simulink model "Bicopter"  (R2025a)
settings: Solver=VariableStepAuto  StartTime=0.0  StopTime=10.0  RelTol=1e-3
values from neighbouring files (symbols this model uses):
  g = 9.81    [biCopter_Variable_script.m]
  initial_states = [initial_position; initial_angles; initial_velocity; initial_ang_velocity]    [biCopter_Variable_script.m]
  Ixx = 0.005    [biCopter_Variable_script.m]
  Iyy = 0.005    [biCopter_Variable_script.m]
  Izz = 0.01    [biCopter_Variable_script.m]
  k_T = 1.5e-6    (= 1.5e-06)    [biCopter_Variable_script.m]
  L = 0.25    [biCopter_Variable_script.m]
  m = 0.5    [biCopter_Variable_script.m]
  max_servo_angle = pi/6    (= 0.523598775598)    [biCopter_Variable_script.m]
  max_thrust_per_motor = 5    [biCopter_Variable_script.m]
  min_servo_angle = -pi/6    (= -0.523598775598)    [biCopter_Variable_script.m]
  min_thrust_per_motor = 0    [biCopter_Variable_script.m]
  tau_motor = 0.05    [biCopter_Variable_script.m]
libraries: slpidlib x4
settings Model: Creator=adity  LastModifiedBy=adity

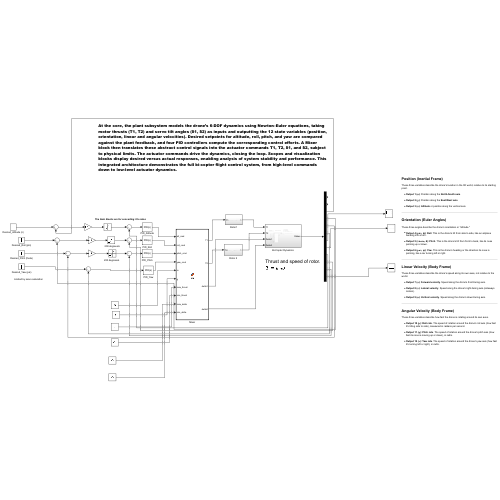
[thumbnail: Simulink's stored preview of the top-level diagram]
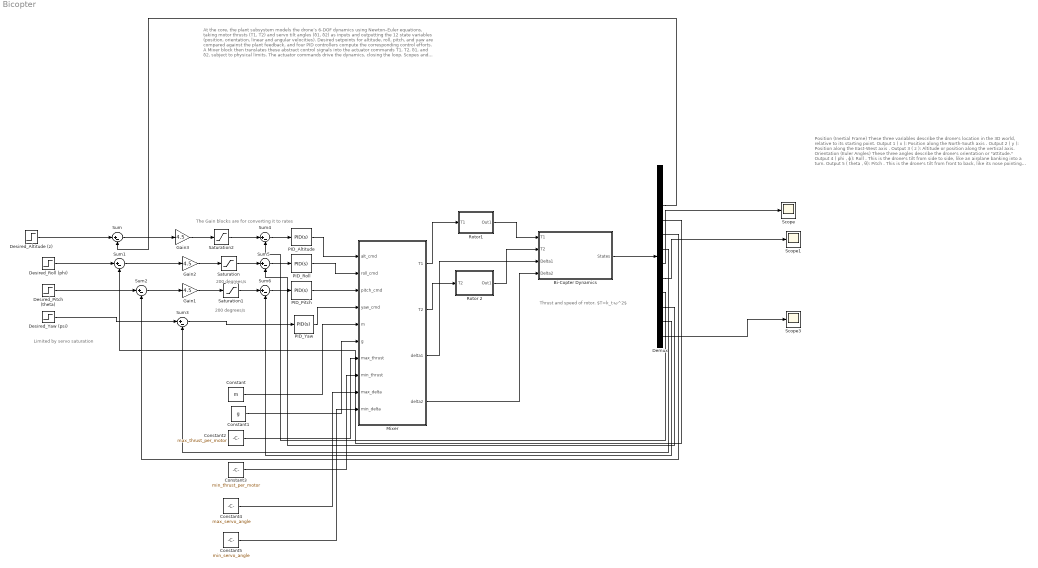
== system Bicopter ==
  note: Limited by servo saturation
  note: 200 degrees/s
  note: The Gain blocks are for converting it to rates
  note: Position (Inertial Frame)
      | These three variables describe the drone's location in the 3D world, relative to its starting point.
      | Output 1 ( x ): Position along the North-South axis .
      | Output 2 ( y ): Position along the East-West axis .
      | Output 3 ( z ): Altitude or position along the vertical axis.
      | Orientation (Euler Angles)
      | These three angles describe the drone's orientation or "attitude."
      | Output 4 ( phi , ϕ): Roll . This is the drone's tilt from side to side, like an airplane banking into a turn.
      | Output 5 ( theta , θ): Pitch . This is the drone's tilt from front to back, like its nose pointing up or down.
      | Output 6 ( psi , ψ): Yaw . This is the drone's heading or the direction its nose is pointing, like a car turning left or right.
      | Linear Velocity (Body Frame)
      | These three variables describe the drone's speed along its own axes, not relative to the world.
      | Output 7 ( u ): Forward velocity . Speed along the drone's front-facing axis.
      | Output 8 ( v ): Lateral velocity . Speed along the drone's right-facing axis (sideways motion).
      | Output 9 ( w ): Vertical velocity . Speed along the drone's down-facing axis.
      | Angular Velocity (Body Frame)
      | These three variables describe how fast the drone is rotating around its own axes.
      | Output 10 ( p ): Roll rate . The speed of rotation around the drone's roll axis (how fast it's tilting side to side), measured in radians per second.
      | Output 11 ( q ): Pitch rate . The speed of rotation around the drone's pitch axis (how fast its nose is moving up or down), in rad/s.
      | Output 12 ( r ): Yaw rate . The speed of rotation around the drone's yaw axis (how fast it's turning left or right), in rad/s.
  note: Thrust and speed of rotor.
      | $T=k_t​⋅ω^2$
  note: At the core, the plant subsystem models the drone’s 6-DOF dynamics using Newton–Euler equations, taking motor thrusts (T1, T2) and servo tilt angles (δ1, δ2) as inputs and outputting the 12 state variables (position, orientation, linear and angular velocities). Desired setpoints for altitude, roll, pitch, and yaw are compared against the plant feedback, and four PID controllers compute the corresponding control efforts. A Mixer block then translates these abstract control signals into the actuator commands T1, T2, δ1, and δ2, subject to physical limits. The actuator commands drive the dynamics, closing the loop. Scopes and visualization blocks display desired versus actual responses, enabling analysis of system stability and performance. This integrated architecture demonstrates the full bi-copter flight control system, from high-level commands down to low-level actuator dynamics.
  note: 200 degrees/s
  Bi-Copter Dynamics : Subsystem
  Constant : Constant  Value=m
  Constant1 : Constant  Value=g
  Constant2 : Constant  Value=max_thrust_per_motor
  Constant3 : Constant  Value=min_thrust_per_motor
  Constant4 : Constant  Value=max_servo_angle
  Constant5 : Constant  Value=min_servo_angle
  Demux : Demux  Outputs=12
  Desired_Altitude (z) : Step  Time=0  After=500  SampleTime=0
  Desired_Pitch (theta) : Step  Time=0  After=0.5  SampleTime=0
  Desired_Roll (phi) : Step  Time=0  After=10  SampleTime=0
  Desired_Yaw (psi) : Step  Time=0  After=2.3  SampleTime=0
  Gain1 : Gain  Gain=4.5
  Gain2 : Gain  Gain=4.5
  Gain3 : Gain  Gain=4.5
  Mixer : MATLAB Function  TreatAsAtomicUnit=on
  PID_Altitude : slpidlib/PID Controller  Controller=PID  Form=Parallel  TimeDomain=Continuous-time  UseExternalTs=off  SampleTime=-1  IntegratorMethod=Forward Euler  FilterMethod=Forward Euler  ControllerParametersSource=internal  P=1  I=1  UseKiTs=off  D=0  UseExternalDerivativeSource=off  N=100  UseFilter=on  TunerSelectOption=Transfer Function Based (PID Tuner App)  InitialConditionSource=internal  InitialConditionForIntegrator=0  InitialConditionForFilter=0  DifferentiatorICPrevScaledInput=0  ExternalReset=none  TrackingMode=off  Kt=1  LimitOutput=off  SatLimitsSource=internal  UpperSaturationLimit=inf  LowerSaturationLimit=-inf  LinearizeAsGain=on  AntiWindupMode=none  Kb=1  LimitIntegrator=off  UpperIntegratorSaturationLimit=inf  LowerIntegratorSaturationLimit=-inf  POutMin=[]  POutMax=[]  IOutMin=[]  IOutMax=[]  DOutMin=[]  DOutMax=[]  NOutMin=[]  NOutMax=[]  SumOutMin=[]  SumOutMax=[]  SaturationOutMin=[]  SaturationOutMax=[]  PParamMin=[]  PParamMax=[]  IParamMin=[]  IParamMax=[]  DParamMin=[]  DParamMax=[]  NParamMin=[]  NParamMax=[]  KbParamMin=[]  KbParamMax=[]  KtParamMin=[]  KtParamMax=[]  KbOutMin=[]  KbOutMax=[]  KtOutMin=[]  KtOutMax=[]  IntegratorOutMin=[]  IntegratorOutMax=[]  FilterOutMin=[]  FilterOutMax=[]  SumI1OutMin=[]  SumI1OutMax=[]  SumI2OutMin=[]  SumI2OutMax=[]  SumI3OutMin=[]  SumI3OutMax=[]  SumI4OutMin=[]  SumI4OutMax=[]  SumDOutMin=[]  SumDOutMax=[]  DifferentiatorOutMin=[]  DifferentiatorOutMax=[]  FilterDiffOutCoefMin=[]  FilterDiffOutCoefMax=[]  ReciprocalOutMin=[]  ReciprocalOutMax=[]  SumDenOutMin=[]  SumDenOutMax=[]  SumNumOutMin=[]  SumNumOutMax=[]  DivideOutMin=[]  DivideOutMax=[]  UdiffTsProdOutMin=[]  UdiffTsProdOutMax=[]  NTsProdOutMin=[]  NTsProdOutMax=[]  UintegralTsProdOutMin=[]  UintegralTsProdOutMax=[]  UngainTsProdOutMin=[]  UngainTsProdOutMax=[]  ClampingZeroOutDataTypeStr=Inherit: Inherit via back propagation  ClampingZeroOutMin=[]  ClampingZeroOutMax=[]  FilterDenConstantOutDataTypeStr=Inherit: Inherit via back propagation  FilterDenConstantOutMin=[]  FilterDenConstantOutMax=[]  PCopyOutDataTypeStr=Inherit: Inherit via back propagation  PCopyOutMin=[]  PCopyOutMax=[]  NCopyOutDataTypeStr=Inherit: Inherit via back propagation  NCopyOutMin=[]  NCopyOutMax=[]  IntegratorContinuousStateAttributes=''  IntegratorStateMustResolveToSignalObject=off  IntegratorRTWStateStorageClass=Auto  FilterContinuousStateAttributes=''  FilterStateMustResolveToSignalObject=off  FilterRTWStateStorageClass=Auto  ParallelPVariant=InternalParameters  IdealPVariant=Disabled  IVariant=InternalParameters  DVariant=InternalParameters  IntegratorVariant=Continuous  SatVariant=Disabled  AWVariant=Passthrough  PCopyVariant=Disabled  TRVariant=Disabled  FdbkBlocksVariant=Forward  IdealPFdbkVariant=Disabled  SatFdbkVariant=Disabled  DerivativeFilterVariant=ContFilter  NVariant=InternalParameters  NCopyVariant=Disabled  FilterICVariant=InternalICsFilter  IntegratorICVariant=InternalICs  ExternalResetVariant=Disabled  TRSumVariant=Passthrough  SumFdbkVariant=Disabled  SumVariant=Sum_PID  TsampFilterVariant=InternalTs  TsampNgainVariant=Passthrough  TsampIntegralVariant=Disabled_SignalSpec  ExternalSaturationOutDataTypeStr=Inherit: Same as second input  DerivativeSourceVariant=ErrorSignal  PreIntVariant=InternalPreInt
  PID_Pitch : slpidlib/PID Controller  Controller=PID  Form=Parallel  TimeDomain=Continuous-time  UseExternalTs=off  SampleTime=-1  IntegratorMethod=Forward Euler  FilterMethod=Forward Euler  ControllerParametersSource=internal  P=1  I=1  UseKiTs=off  D=0  UseExternalDerivativeSource=off  N=100  UseFilter=on  TunerSelectOption=Transfer Function Based (PID Tuner App)  InitialConditionSource=internal  InitialConditionForIntegrator=0  InitialConditionForFilter=0  DifferentiatorICPrevScaledInput=0  ExternalReset=none  TrackingMode=off  Kt=1  LimitOutput=off  SatLimitsSource=internal  UpperSaturationLimit=inf  LowerSaturationLimit=-inf  LinearizeAsGain=on  AntiWindupMode=none  Kb=1  LimitIntegrator=off  UpperIntegratorSaturationLimit=inf  LowerIntegratorSaturationLimit=-inf  POutMin=[]  POutMax=[]  IOutMin=[]  IOutMax=[]  DOutMin=[]  DOutMax=[]  NOutMin=[]  NOutMax=[]  SumOutMin=[]  SumOutMax=[]  SaturationOutMin=[]  SaturationOutMax=[]  PParamMin=[]  PParamMax=[]  IParamMin=[]  IParamMax=[]  DParamMin=[]  DParamMax=[]  NParamMin=[]  NParamMax=[]  KbParamMin=[]  KbParamMax=[]  KtParamMin=[]  KtParamMax=[]  KbOutMin=[]  KbOutMax=[]  KtOutMin=[]  KtOutMax=[]  IntegratorOutMin=[]  IntegratorOutMax=[]  FilterOutMin=[]  FilterOutMax=[]  SumI1OutMin=[]  SumI1OutMax=[]  SumI2OutMin=[]  SumI2OutMax=[]  SumI3OutMin=[]  SumI3OutMax=[]  SumI4OutMin=[]  SumI4OutMax=[]  SumDOutMin=[]  SumDOutMax=[]  DifferentiatorOutMin=[]  DifferentiatorOutMax=[]  FilterDiffOutCoefMin=[]  FilterDiffOutCoefMax=[]  ReciprocalOutMin=[]  ReciprocalOutMax=[]  SumDenOutMin=[]  SumDenOutMax=[]  SumNumOutMin=[]  SumNumOutMax=[]  DivideOutMin=[]  DivideOutMax=[]  UdiffTsProdOutMin=[]  UdiffTsProdOutMax=[]  NTsProdOutMin=[]  NTsProdOutMax=[]  UintegralTsProdOutMin=[]  UintegralTsProdOutMax=[]  UngainTsProdOutMin=[]  UngainTsProdOutMax=[]  ClampingZeroOutDataTypeStr=Inherit: Inherit via back propagation  ClampingZeroOutMin=[]  ClampingZeroOutMax=[]  FilterDenConstantOutDataTypeStr=Inherit: Inherit via back propagation  FilterDenConstantOutMin=[]  FilterDenConstantOutMax=[]  PCopyOutDataTypeStr=Inherit: Inherit via back propagation  PCopyOutMin=[]  PCopyOutMax=[]  NCopyOutDataTypeStr=Inherit: Inherit via back propagation  NCopyOutMin=[]  NCopyOutMax=[]  IntegratorContinuousStateAttributes=''  IntegratorStateMustResolveToSignalObject=off  IntegratorRTWStateStorageClass=Auto  FilterContinuousStateAttributes=''  FilterStateMustResolveToSignalObject=off  FilterRTWStateStorageClass=Auto  ParallelPVariant=InternalParameters  IdealPVariant=Disabled  IVariant=InternalParameters  DVariant=InternalParameters  IntegratorVariant=Continuous  SatVariant=Disabled  AWVariant=Passthrough  PCopyVariant=Disabled  TRVariant=Disabled  FdbkBlocksVariant=Forward  IdealPFdbkVariant=Disabled  SatFdbkVariant=Disabled  DerivativeFilterVariant=ContFilter  NVariant=InternalParameters  NCopyVariant=Disabled  FilterICVariant=InternalICsFilter  IntegratorICVariant=InternalICs  ExternalResetVariant=Disabled  TRSumVariant=Passthrough  SumFdbkVariant=Disabled  SumVariant=Sum_PID  TsampFilterVariant=InternalTs  TsampNgainVariant=Passthrough  TsampIntegralVariant=Disabled_SignalSpec  ExternalSaturationOutDataTypeStr=Inherit: Same as second input  DerivativeSourceVariant=ErrorSignal  PreIntVariant=InternalPreInt
  PID_Roll : slpidlib/PID Controller  Controller=PID  Form=Parallel  TimeDomain=Continuous-time  UseExternalTs=off  SampleTime=-1  IntegratorMethod=Forward Euler  FilterMethod=Forward Euler  ControllerParametersSource=internal  P=1  I=1  UseKiTs=off  D=0  UseExternalDerivativeSource=off  N=100  UseFilter=on  TunerSelectOption=Transfer Function Based (PID Tuner App)  InitialConditionSource=internal  InitialConditionForIntegrator=0  InitialConditionForFilter=0  DifferentiatorICPrevScaledInput=0  ExternalReset=none  TrackingMode=off  Kt=1  LimitOutput=off  SatLimitsSource=internal  UpperSaturationLimit=inf  LowerSaturationLimit=-inf  LinearizeAsGain=on  AntiWindupMode=none  Kb=1  LimitIntegrator=off  UpperIntegratorSaturationLimit=inf  LowerIntegratorSaturationLimit=-inf  POutMin=[]  POutMax=[]  IOutMin=[]  IOutMax=[]  DOutMin=[]  DOutMax=[]  NOutMin=[]  NOutMax=[]  SumOutMin=[]  SumOutMax=[]  SaturationOutMin=[]  SaturationOutMax=[]  PParamMin=[]  PParamMax=[]  IParamMin=[]  IParamMax=[]  DParamMin=[]  DParamMax=[]  NParamMin=[]  NParamMax=[]  KbParamMin=[]  KbParamMax=[]  KtParamMin=[]  KtParamMax=[]  KbOutMin=[]  KbOutMax=[]  KtOutMin=[]  KtOutMax=[]  IntegratorOutMin=[]  IntegratorOutMax=[]  FilterOutMin=[]  FilterOutMax=[]  SumI1OutMin=[]  SumI1OutMax=[]  SumI2OutMin=[]  SumI2OutMax=[]  SumI3OutMin=[]  SumI3OutMax=[]  SumI4OutMin=[]  SumI4OutMax=[]  SumDOutMin=[]  SumDOutMax=[]  DifferentiatorOutMin=[]  DifferentiatorOutMax=[]  FilterDiffOutCoefMin=[]  FilterDiffOutCoefMax=[]  ReciprocalOutMin=[]  ReciprocalOutMax=[]  SumDenOutMin=[]  SumDenOutMax=[]  SumNumOutMin=[]  SumNumOutMax=[]  DivideOutMin=[]  DivideOutMax=[]  UdiffTsProdOutMin=[]  UdiffTsProdOutMax=[]  NTsProdOutMin=[]  NTsProdOutMax=[]  UintegralTsProdOutMin=[]  UintegralTsProdOutMax=[]  UngainTsProdOutMin=[]  UngainTsProdOutMax=[]  ClampingZeroOutDataTypeStr=Inherit: Inherit via back propagation  ClampingZeroOutMin=[]  ClampingZeroOutMax=[]  FilterDenConstantOutDataTypeStr=Inherit: Inherit via back propagation  FilterDenConstantOutMin=[]  FilterDenConstantOutMax=[]  PCopyOutDataTypeStr=Inherit: Inherit via back propagation  PCopyOutMin=[]  PCopyOutMax=[]  NCopyOutDataTypeStr=Inherit: Inherit via back propagation  NCopyOutMin=[]  NCopyOutMax=[]  IntegratorContinuousStateAttributes=''  IntegratorStateMustResolveToSignalObject=off  IntegratorRTWStateStorageClass=Auto  FilterContinuousStateAttributes=''  FilterStateMustResolveToSignalObject=off  FilterRTWStateStorageClass=Auto  ParallelPVariant=InternalParameters  IdealPVariant=Disabled  IVariant=InternalParameters  DVariant=InternalParameters  IntegratorVariant=Continuous  SatVariant=Disabled  AWVariant=Passthrough  PCopyVariant=Disabled  TRVariant=Disabled  FdbkBlocksVariant=Forward  IdealPFdbkVariant=Disabled  SatFdbkVariant=Disabled  DerivativeFilterVariant=ContFilter  NVariant=InternalParameters  NCopyVariant=Disabled  FilterICVariant=InternalICsFilter  IntegratorICVariant=InternalICs  ExternalResetVariant=Disabled  TRSumVariant=Passthrough  SumFdbkVariant=Disabled  SumVariant=Sum_PID  TsampFilterVariant=InternalTs  TsampNgainVariant=Passthrough  TsampIntegralVariant=Disabled_SignalSpec  ExternalSaturationOutDataTypeStr=Inherit: Same as second input  DerivativeSourceVariant=ErrorSignal  PreIntVariant=InternalPreInt
  PID_Yaw : slpidlib/PID Controller  Controller=PID  Form=Parallel  TimeDomain=Continuous-time  UseExternalTs=off  SampleTime=-1  IntegratorMethod=Forward Euler  FilterMethod=Forward Euler  ControllerParametersSource=internal  P=1  I=1  UseKiTs=off  D=0  UseExternalDerivativeSource=off  N=100  UseFilter=on  TunerSelectOption=Transfer Function Based (PID Tuner App)  InitialConditionSource=internal  InitialConditionForIntegrator=0  InitialConditionForFilter=0  DifferentiatorICPrevScaledInput=0  ExternalReset=none  TrackingMode=off  Kt=1  LimitOutput=off  SatLimitsSource=internal  UpperSaturationLimit=inf  LowerSaturationLimit=-inf  LinearizeAsGain=on  AntiWindupMode=none  Kb=1  LimitIntegrator=off  UpperIntegratorSaturationLimit=inf  LowerIntegratorSaturationLimit=-inf  POutMin=[]  POutMax=[]  IOutMin=[]  IOutMax=[]  DOutMin=[]  DOutMax=[]  NOutMin=[]  NOutMax=[]  SumOutMin=[]  SumOutMax=[]  SaturationOutMin=[]  SaturationOutMax=[]  PParamMin=[]  PParamMax=[]  IParamMin=[]  IParamMax=[]  DParamMin=[]  DParamMax=[]  NParamMin=[]  NParamMax=[]  KbParamMin=[]  KbParamMax=[]  KtParamMin=[]  KtParamMax=[]  KbOutMin=[]  KbOutMax=[]  KtOutMin=[]  KtOutMax=[]  IntegratorOutMin=[]  IntegratorOutMax=[]  FilterOutMin=[]  FilterOutMax=[]  SumI1OutMin=[]  SumI1OutMax=[]  SumI2OutMin=[]  SumI2OutMax=[]  SumI3OutMin=[]  SumI3OutMax=[]  SumI4OutMin=[]  SumI4OutMax=[]  SumDOutMin=[]  SumDOutMax=[]  DifferentiatorOutMin=[]  DifferentiatorOutMax=[]  FilterDiffOutCoefMin=[]  FilterDiffOutCoefMax=[]  ReciprocalOutMin=[]  ReciprocalOutMax=[]  SumDenOutMin=[]  SumDenOutMax=[]  SumNumOutMin=[]  SumNumOutMax=[]  DivideOutMin=[]  DivideOutMax=[]  UdiffTsProdOutMin=[]  UdiffTsProdOutMax=[]  NTsProdOutMin=[]  NTsProdOutMax=[]  UintegralTsProdOutMin=[]  UintegralTsProdOutMax=[]  UngainTsProdOutMin=[]  UngainTsProdOutMax=[]  ClampingZeroOutDataTypeStr=Inherit: Inherit via back propagation  ClampingZeroOutMin=[]  ClampingZeroOutMax=[]  FilterDenConstantOutDataTypeStr=Inherit: Inherit via back propagation  FilterDenConstantOutMin=[]  FilterDenConstantOutMax=[]  PCopyOutDataTypeStr=Inherit: Inherit via back propagation  PCopyOutMin=[]  PCopyOutMax=[]  NCopyOutDataTypeStr=Inherit: Inherit via back propagation  NCopyOutMin=[]  NCopyOutMax=[]  IntegratorContinuousStateAttributes=''  IntegratorStateMustResolveToSignalObject=off  IntegratorRTWStateStorageClass=Auto  FilterContinuousStateAttributes=''  FilterStateMustResolveToSignalObject=off  FilterRTWStateStorageClass=Auto  ParallelPVariant=InternalParameters  IdealPVariant=Disabled  IVariant=InternalParameters  DVariant=InternalParameters  IntegratorVariant=Continuous  SatVariant=Disabled  AWVariant=Passthrough  PCopyVariant=Disabled  TRVariant=Disabled  FdbkBlocksVariant=Forward  IdealPFdbkVariant=Disabled  SatFdbkVariant=Disabled  DerivativeFilterVariant=ContFilter  NVariant=InternalParameters  NCopyVariant=Disabled  FilterICVariant=InternalICsFilter  IntegratorICVariant=InternalICs  ExternalResetVariant=Disabled  TRSumVariant=Passthrough  SumFdbkVariant=Disabled  SumVariant=Sum_PID  TsampFilterVariant=InternalTs  TsampNgainVariant=Passthrough  TsampIntegralVariant=Disabled_SignalSpec  ExternalSaturationOutDataTypeStr=Inherit: Same as second input  DerivativeSourceVariant=ErrorSignal  PreIntVariant=InternalPreInt
  Rotor 2 : Subsystem
  Rotor1 : Subsystem
  Saturation : Saturate  UpperLimit=3.49  LowerLimit=-3.49
  Saturation1 : Saturate  UpperLimit=3.49  LowerLimit=-3.49
  Saturation2 : Saturate  UpperLimit=1  LowerLimit=-1
  Scope : Scope
      settings: ActiveDisplayYMinimum=-88.144858424605019  ActiveDisplayYMaximum=88.937365144154228
  Scope1 : Scope
      settings: ActiveDisplayYMinimum=-88.7441974939224  ActiveDisplayYMaximum=88.748617026885341
  Scope3 : Scope
      settings: ActiveDisplayYMinimum=-106.7500117856095  ActiveDisplayYMaximum=32.830412504409331  DataLoggingVariableName=ScopeData3
  Sum{,1..6} (7 alike) : Sum  Inputs=|+-
  wires:
  Desired_Altitude (z)/1 -> Sum/1
  Desired_Roll (phi)/1 -> Sum1/1
  Desired_Pitch (theta)/1 -> Sum2/1
  Desired_Yaw (psi)/1 -> Sum3/1
  PID_Altitude/1 -> Mixer/1(alt_cmd)
  PID_Roll/1 -> Mixer/2(roll_cmd)
  PID_Pitch/1 -> Mixer/3(pitch_cmd)
  PID_Yaw/1 -> Mixer/4(yaw_cmd)
  Mixer/3(delta1) -> Bi-Copter Dynamics/3(Delta1)
  Mixer/4(delta2) -> Bi-Copter Dynamics/4(Delta2)
  Bi-Copter Dynamics/1(States) -> Demux/1
  Demux/3 -> Sum/2
  Demux/5 -> Sum2/2
  Demux/6 -> Sum3/2
  Demux/4 -> Sum1/2
  Constant/1 -> Mixer/5(m)
  Constant1/1 -> Mixer/6(g)
  Constant2/1 -> Mixer/7(max_thrust)
  Constant3/1 -> Mixer/8(min_thrust)
  Constant4/1 -> Mixer/9(max_delta)
  Constant5/1 -> Mixer/10(min_delta)
  Mixer/1(T1) -> Rotor1/1(T1)
  Rotor1/1(Out1) -> Bi-Copter Dynamics/1(T1)
  Mixer/2(T2) -> Rotor 2/1(T2)
  Rotor 2/1(Out1) -> Bi-Copter Dynamics/2(T2)
  Sum/1 -> Gain3/1
  Sum1/1 -> Gain2/1
  Sum2/1 -> Gain1/1
  Sum3/1 -> PID_Yaw/1
  Sum4/1 -> PID_Altitude/1
  Sum5/1 -> PID_Roll/1
  Sum6/1 -> PID_Pitch/1
  Demux/9 -> Sum4/2
  Demux/10 -> Sum5/2
  Demux/11 -> Sum6/2
  Demux/7 -> Scope/1
  Demux/8 -> Scope1/1
  Demux/12 -> Scope3/1
  Gain1/1 -> Saturation1/1
  Saturation1/1 -> Sum6/1
  Gain2/1 -> Saturation/1
  Saturation/1 -> Sum5/1
  Gain3/1 -> Saturation2/1
  Saturation2/1 -> Sum4/1

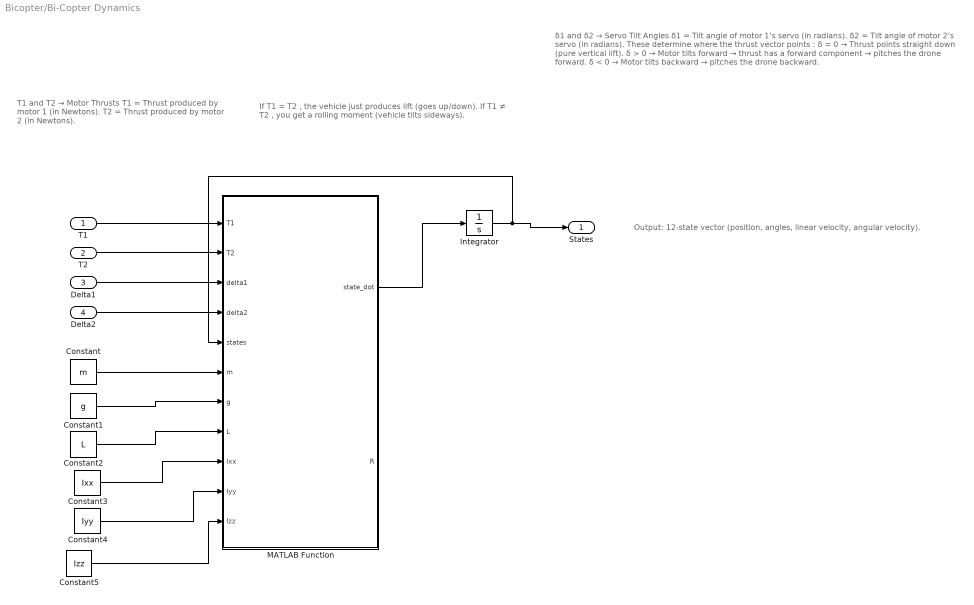
== system Bicopter/Bi-Copter Dynamics ==
  note: Output: 12-state vector (position, angles, linear velocity, angular velocity).
  note: δ1 and δ2 → Servo Tilt Angles
      | δ1 = Tilt angle of motor 1’s servo (in radians).
      | δ2 = Tilt angle of motor 2’s servo (in radians).
      | These determine where the thrust vector points :
      | δ = 0 → Thrust points straight down (pure vertical lift).
      | δ > 0 → Motor tilts forward → thrust has a forward component → pitches the drone forward.
      | δ < 0 → Motor tilts backward → pitches the drone backward.
  note: If T1 = T2 , the vehicle just produces lift (goes up/down).
      | If T1 ≠ T2 , you get a rolling moment (vehicle tilts sideways).
  note: T1 and T2 → Motor Thrusts
      | T1 = Thrust produced by motor 1 (in Newtons).
      | T2 = Thrust produced by motor 2 (in Newtons).
  T1 : Inport
  T2 : Inport  Port=2
  Delta1 : Inport  Port=3
  Delta2 : Inport  Port=4
  Constant : Constant  Value=m
  Constant1 : Constant  Value=g
  Constant2 : Constant  Value=L
  Constant3 : Constant  Value=Ixx
  Constant4 : Constant  Value=Iyy
  Constant5 : Constant  Value=Izz
  Integrator : Integrator  InitialCondition=initial_states
  MATLAB Function : MATLAB Function  TreatAsAtomicUnit=on
  States : Outport
  wires:
  MATLAB Function/1(state_dot) -> Integrator/1
  Integrator/1 -> MATLAB Function/5(states), States/1
  T1/1 -> MATLAB Function/1(T1)
  T2/1 -> MATLAB Function/2(T2)
  Delta1/1 -> MATLAB Function/3(delta1)
  Delta2/1 -> MATLAB Function/4(delta2)
  Constant/1 -> MATLAB Function/6(m)
  Constant1/1 -> MATLAB Function/7(g)
  Constant2/1 -> MATLAB Function/8(L)
  Constant3/1 -> MATLAB Function/9(Ixx)
  Constant4/1 -> MATLAB Function/10(Iyy)
  Constant5/1 -> MATLAB Function/11(Izz)

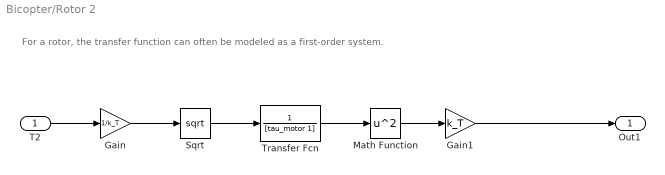
== system Bicopter/Rotor 2 ==
  note: For a rotor, the transfer function can often be modeled as a first-order system.
  T2 : Inport
  Gain : Gain  Gain=1/k_T
  Gain1 : Gain  Gain=k_T
  Math Function : Math  Operator=square
  Sqrt : Sqrt
  Transfer Fcn : TransferFcn  Denominator=[tau_motor 1]
  Out1 : Outport
  wires:
  T2/1 -> Gain/1
  Gain/1 -> Sqrt/1
  Sqrt/1 -> Transfer Fcn/1
  Transfer Fcn/1 -> Math Function/1
  Math Function/1 -> Gain1/1
  Gain1/1 -> Out1/1

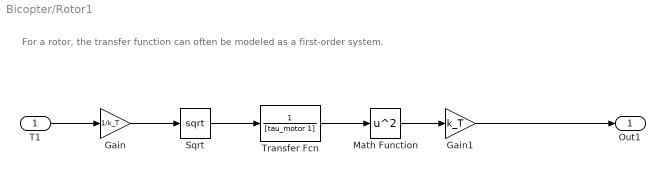
== system Bicopter/Rotor1 ==
  note: For a rotor, the transfer function can often be modeled as a first-order system.
  T1 : Inport
  Gain : Gain  Gain=1/k_T
  Gain1 : Gain  Gain=k_T
  Math Function : Math  Operator=square
  Sqrt : Sqrt
  Transfer Fcn : TransferFcn  Denominator=[tau_motor 1]
  Out1 : Outport
  wires:
  T1/1 -> Gain/1
  Gain/1 -> Sqrt/1
  Sqrt/1 -> Transfer Fcn/1
  Transfer Fcn/1 -> Math Function/1
  Math Function/1 -> Gain1/1
  Gain1/1 -> Out1/1

== matlab function Bicopter/Mixer ==
  data: alt_cmd input; T1 output; roll_cmd input; pitch_cmd input; yaw_cmd input; T2 output; delta1 output; delta2 output; m input; g input; max_thrust input; min_thrust input; max_delta input; min_delta input
function [T1, T2, delta1, delta2] = fcn(alt_cmd, roll_cmd, pitch_cmd, yaw_cmd, m, g, max_thrust, min_thrust, max_delta, min_delta)
base_thrust = m*g;
total_thrust = base_thrust + alt_cmd;
T1 = total_thrust/2 - roll_cmd;
T2 = total_thrust/2 + roll_cmd;
delta1 = pitch_cmd - yaw_cmd;
delta2 = pitch_cmd + yaw_cmd;
T1 = max(min_thrust, min(T1, max_thrust));
T2 = max(min_thrust, min(T2, max_thrust));
delta1 = max(min_delta, min(delta1, max_delta));
delta2 = max(min_delta, min(delta2, max_delta));
end

== matlab function Bicopter/Bi-Copter Dynamics/MATLAB Function ==
  data: T1 input; state_dot output; T2 input; delta1 input; delta2 input; states input; R output; m input; g input; L input; Ixx input; Iyy input; Izz input
function [state_dot, R] = fcn(T1, T2, delta1, delta2, states, m, g, L, Ixx, Iyy, Izz)
phi=states(4); theta=states(5); psi=states(6); 
u=states(7); v=states(8); w=states(9);
p=states(10); q=states(11); r=states(12);
cphi = cos(phi); sphi = sin(phi);
cthe = cos(theta); sthe = sin(theta);
cpsi = cos(psi); spsi = sin(psi);
R = [cthe*cpsi, sphi*sthe*cpsi-cphi*spsi, cphi*sthe*cpsi+sphi*spsi;
     cthe*spsi, sphi*sthe*spsi+cphi*cpsi, cphi*sthe*spsi-sphi*cpsi;
     -sthe,     sphi*cthe,              cphi*cthe];
Thrust_forces = [(T1*sin(delta1) + T2*sin(delta2));
                 0;
                 -(T1*cos(delta1) + T2*cos(delta2))];
Gravity_forces = R' * [0; 0; m*g];
uvw_dot = (1/m)*(Gravity_forces + Thrust_forces) - cross([p;q;r], [u;v;w]);
Torques = [L * (T1*cos(delta1) - T2*cos(delta2));
           L * (T1*sin(delta1) - T2*sin(delta2));
           L * (T1*sin(delta1) + T2*sin(delta2))]; 
pqr_dot = [1/Ixx; 1/Iyy; 1/Izz] .* (Torques - cross([p;q;r], [Ixx*p; Iyy*q; Izz*r]));
angle_dot = [1, sphi*tan(theta), cphi*tan(theta);
             0, cphi,            -sphi;
             0, sphi/cthe,       cphi/cthe] * [p;q;r];
pos_dot = R * [u;v;w];
state_dot = [pos_dot; angle_dot; uvw_dot; pqr_dot];
end
